simulink model "diplom_model"  (R2015a)
settings: Solver=ode45  StartTime=0.0  StopTime=10.0  RelTol=1e-3
libraries: fuzblock x2, simulink_need_slupdate x2
settings Model: Creator=Vlad  LastModifiedBy=Vlad

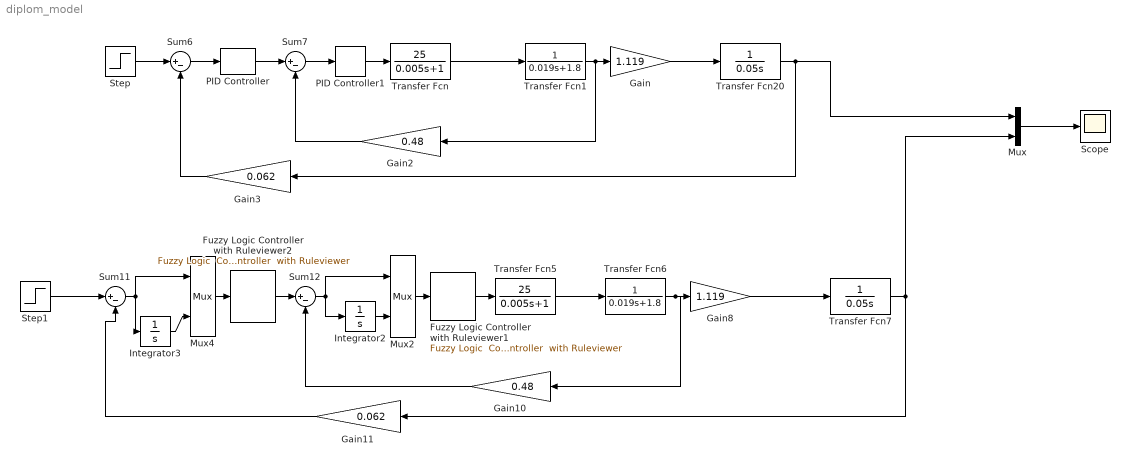
== system diplom_model ==
  Fuzzy Logic Controller with Ruleviewer1 : fuzblock/Fuzzy Logic  Controller  with Ruleviewer  fismatrix=fuzzy1  Ts=1
  Fuzzy Logic Controller with Ruleviewer2 : fuzblock/Fuzzy Logic  Controller  with Ruleviewer  fismatrix=fuzzy2  Ts=1
  Gain : Gain  Gain=1.119  SaturateOnIntegerOverflow=on  OutDataTypeStr=Inherit: Same as input  ParamDataTypeStr=Inherit: Same as input
  Gain10 : Gain  Gain=0.48  SaturateOnIntegerOverflow=on  OutDataTypeStr=Inherit: Same as input  ParamDataTypeStr=Inherit: Same as input
  Gain11 : Gain  Gain=0.062  SaturateOnIntegerOverflow=on  OutDataTypeStr=Inherit: Same as input  ParamDataTypeStr=Inherit: Same as input
  Gain2 : Gain  Gain=0.48  SaturateOnIntegerOverflow=on  OutDataTypeStr=Inherit: Same as input  ParamDataTypeStr=Inherit: Same as input
  Gain3 : Gain  Gain=0.062  SaturateOnIntegerOverflow=on  OutDataTypeStr=Inherit: Same as input  ParamDataTypeStr=Inherit: Same as input
  Gain8 : Gain  Gain=1.119  SaturateOnIntegerOverflow=on  OutDataTypeStr=Inherit: Same as input  ParamDataTypeStr=Inherit: Same as input
  Integrator2 : Integrator
  Integrator3 : Integrator
  Mux : Mux  Inputs=2
  Mux2 : Mux  Inputs=2
  Mux4 : Mux  Inputs=2
  PID Controller : simulink_need_slupdate/PID Controller  P=6.26  I=313.13  D=0
  PID Controller1 : simulink_need_slupdate/PID Controller  P=0.165  I=14.99  D=0
  Scope : Scope
      settings: TimeRange=0.007027351338174004  YMin=111.3259781553876  YMax=114.7012118016133
  Step : Step  Time=0  After=6.88  SampleTime=0
  Step1 : Step  Time=0  After=10  SampleTime=0
  Sum{6..7,11..12} (4 alike) : Sum  Inputs=|+-  SaturateOnIntegerOverflow=on
  Transfer Fcn : TransferFcn  Numerator=[25]  Denominator=[0.005 1]
  Transfer Fcn1 : TransferFcn  Denominator=[0.019 1.8]
  Transfer Fcn20 : TransferFcn  Denominator=[0.05 0]
  Transfer Fcn5 : TransferFcn  Numerator=[25]  Denominator=[0.005 1]
  Transfer Fcn6 : TransferFcn  Denominator=[0.019 1.8]
  Transfer Fcn7 : TransferFcn  Denominator=[0.05 0]
  wires:
  Step/1 -> Sum6/1
  Transfer Fcn/1 -> Transfer Fcn1/1
  Transfer Fcn1/1 -> Gain/1, Gain2/1
  Gain/1 -> Transfer Fcn20/1
  Transfer Fcn20/1 -> Gain3/1, Mux/1
  Gain2/1 -> Sum7/2
  Gain3/1 -> Sum6/2
  Sum6/1 -> PID Controller/1
  Sum7/1 -> PID Controller1/1
  PID Controller/1 -> Sum7/1
  PID Controller1/1 -> Transfer Fcn/1
  Transfer Fcn5/1 -> Transfer Fcn6/1
  Transfer Fcn6/1 -> Gain10/1, Gain8/1
  Gain8/1 -> Transfer Fcn7/1
  Transfer Fcn7/1 -> Mux/2, Gain11/1
  Gain10/1 -> Sum12/2
  Gain11/1 -> Sum11/2
  Fuzzy Logic Controller with Ruleviewer2/1 -> Sum12/1
  Sum12/1 -> Mux2/1, Integrator2/1
  Integrator2/1 -> Mux2/2
  Fuzzy Logic Controller with Ruleviewer1/1 -> Transfer Fcn5/1
  Mux2/1 -> Fuzzy Logic Controller with Ruleviewer1/1
  Integrator3/1 -> Mux4/2
  Mux4/1 -> Fuzzy Logic Controller with Ruleviewer2/1
  Sum11/1 -> Integrator3/1, Mux4/1
  Step1/1 -> Sum11/1
  Mux/1 -> Scope/1
